simulink model "Flight_Test_Augmented_Model"  (R2024a)
settings: Solver=VariableStepAuto  StartTime=0.0  StopTime=55  RelTol=1e-3
undefined symbols (not defined in the file): a_e_tilde_hat_0, a_e_tilde_max, A_p, B_p, B_pT, degradation_switch, epsilon, g, Gamma_a, K_omega, K_p, k_r, K_v, L, Lambda_baseline, Lambda_deg, lambda_hat_0, lambda_max, nu_b_0, Omega_r_0, p_b_i_0, q_0, t_deg, T_max, T_min, tPoints, UAV, wind_switch, x_hat_0
libraries: matrix_library x2, shareduavrstlib x1
settings Model: Creator=Usuario  LastModifiedBy=Usuario

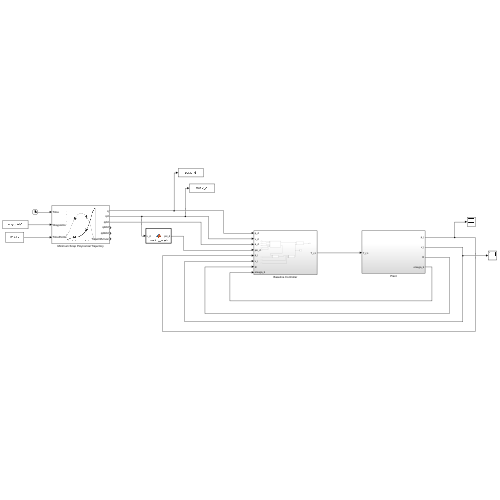
[thumbnail: Simulink's stored preview of the top-level diagram]
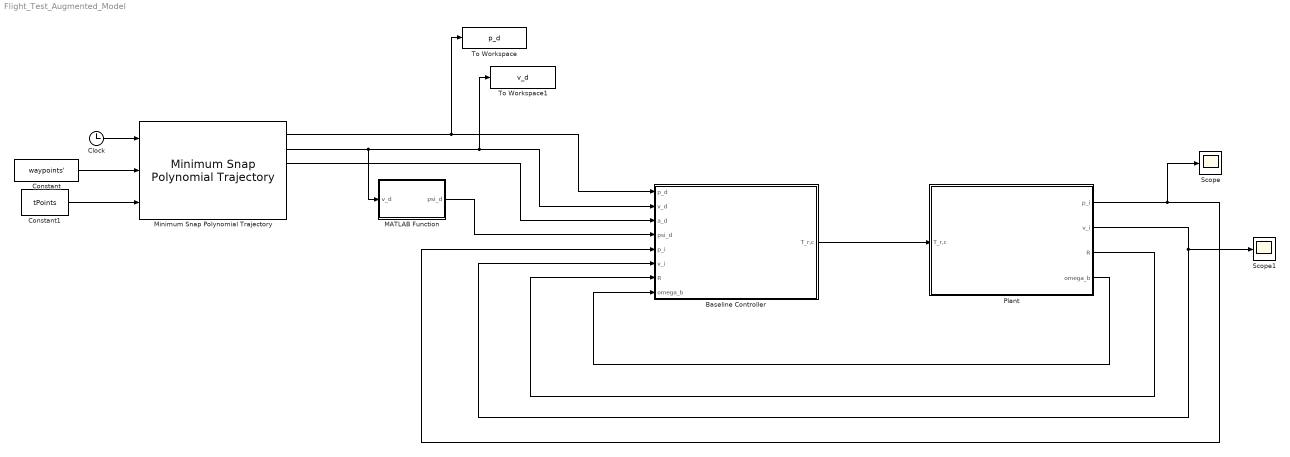
== system Flight_Test_Augmented_Model ==
  Baseline Controller : Subsystem
  Clock : Clock
  Constant : Constant  Value=waypoints'
  Constant1 : Constant  Value=tPoints
  MATLAB Function : MATLAB Function  TreatAsAtomicUnit=on
  Minimum Snap Polynomial Trajectory : shareduavrstlib/Minimum Snap Polynomial Trajectory  ShowBCInputPort=off  ShowPolynomialCoefs=off  ShowStatusOutputPort=off  TimeAllocation=off  TimeWeight=100  MinSegmentTime=0.1  MaxSegmentTime=1  MaxIteration=1500  MaxTime=10  SimulateUsing=Interpreted execution
      settings: LibrarySourceBlock=uavalgslib/Minimum Snap Polynomial Trajectory
  Plant : Subsystem
  Scope : Scope
  Scope1 : Scope
  To Workspace : ToWorkspace  VariableName=p_d  SaveFormat=Timeseries  SampleTime=-1
  To Workspace1 : ToWorkspace  VariableName=v_d  SaveFormat=Timeseries  SampleTime=-1
  wires:
  Baseline Controller/1(T_r,c) -> Plant/1(T_r,c)
  Plant/1(p_i) -> Scope/1, Baseline Controller/5(p_i)
  Plant/2(v_i) -> Baseline Controller/6(v_i), Scope1/1
  Plant/3(R) -> Baseline Controller/7(R)
  Plant/4(omega_b) -> Baseline Controller/8(omega_b)
  Minimum Snap Polynomial Trajectory/3 -> Baseline Controller/3(a_d)
  Clock/1 -> Minimum Snap Polynomial Trajectory/1
  Minimum Snap Polynomial Trajectory/1 -> Baseline Controller/1(p_d), To Workspace/1
  MATLAB Function/1(psi_d) -> Baseline Controller/4(psi_d)
  Constant/1 -> Minimum Snap Polynomial Trajectory/2
  Constant1/1 -> Minimum Snap Polynomial Trajectory/3
  Minimum Snap Polynomial Trajectory/2 -> MATLAB Function/1(v_d), Baseline Controller/2(v_d), To Workspace1/1

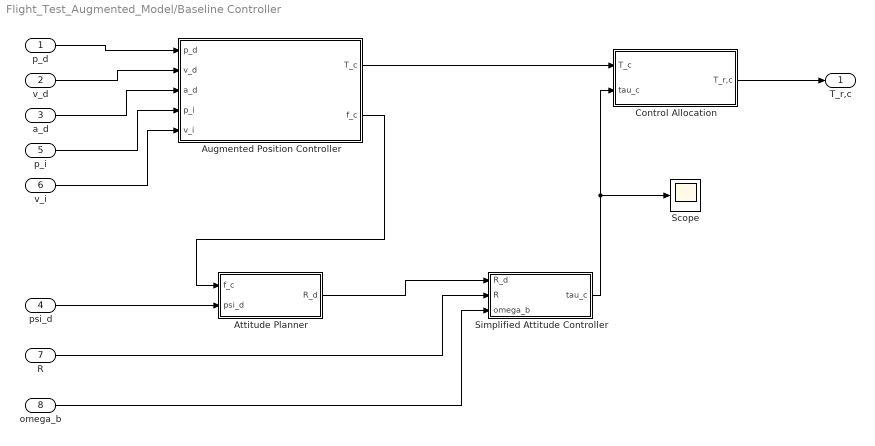
== system Flight_Test_Augmented_Model/Baseline Controller ==
  p_d : Inport
  v_d : Inport  Port=2
  a_d : Inport  Port=3
  psi_d : Inport  Port=4
  p_i : Inport  Port=5
  v_i : Inport  Port=6
  R : Inport  Port=7
  omega_b : Inport  Port=8
  Attitude Planner : Subsystem
  Augmented Position Controller : Subsystem
  Control Allocation : Subsystem
  Scope : Scope
  Simplified Attitude Controller : Subsystem
  T_r,c : Outport
  wires:
  Control Allocation/1(T_r,c) -> T_r,c/1
  p_d/1 -> Augmented Position Controller/1(p_d)
  v_d/1 -> Augmented Position Controller/2(v_d)
  a_d/1 -> Augmented Position Controller/3(a_d)
  Augmented Position Controller/1(T_c) -> Control Allocation/1(T_c)
  psi_d/1 -> Attitude Planner/2(psi_d)
  Augmented Position Controller/2(f_c) -> Attitude Planner/1(f_c)
  Attitude Planner/1(R_d) -> Simplified Attitude Controller/1(R_d)
  Simplified Attitude Controller/1(tau_c) -> Scope/1, Control Allocation/2(tau_c)
  p_i/1 -> Augmented Position Controller/4(p_i)
  v_i/1 -> Augmented Position Controller/5(v_i)
  R/1 -> Simplified Attitude Controller/2(R)
  omega_b/1 -> Simplified Attitude Controller/3(omega_b)

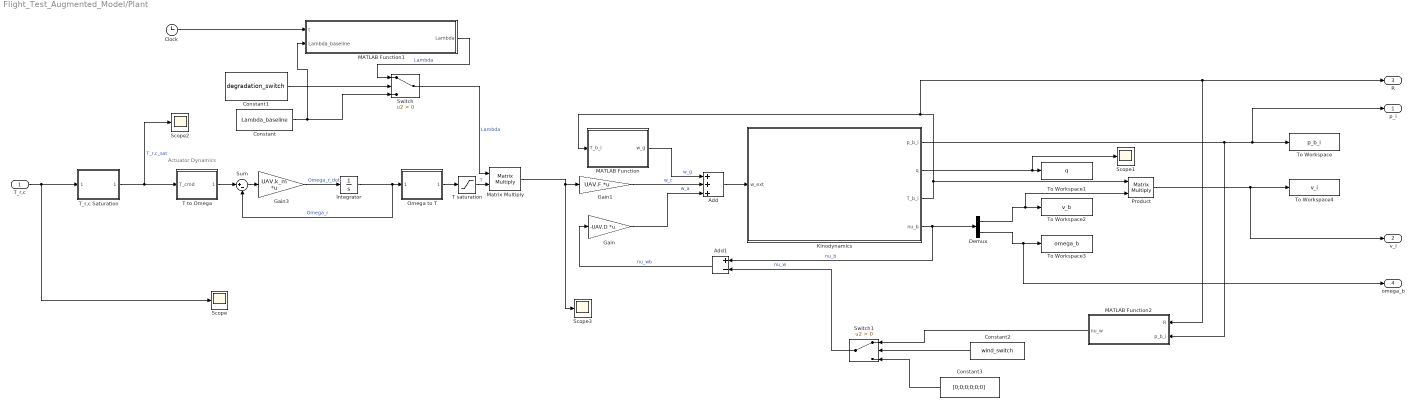
== system Flight_Test_Augmented_Model/Plant ==
  note: Actuator Dynamics
  T_r,c : Inport
  " Omega to T" : MATLAB Function  TreatAsAtomicUnit=on
  " T to Omega" : MATLAB Function  TreatAsAtomicUnit=on
  Add : Sum  Inputs=+++
  Add1 : Sum  Inputs=+-
  Clock : Clock
  Constant : Constant  Value=Lambda_baseline
  Constant1 : Constant  Value=degradation_switch
  Constant2 : Constant  Value=wind_switch
  Constant3 : Constant  Value=[0;0;0;0;0;0]
  Demux : Demux  Outputs=[3 3]
  Gain : Gain  Gain=-UAV.D  Multiplication=Matrix(K*u)
  Gain1 : Gain  Gain=UAV.F  Multiplication=Matrix(K*u)
  Gain3 : Gain  Gain=UAV.k_m  Multiplication=Matrix(K*u)
  Integrator : Integrator  InitialCondition=Omega_r_0
  Kinodynamics : Subsystem
  MATLAB Function : MATLAB Function  TreatAsAtomicUnit=on
  MATLAB Function1 : MATLAB Function  TreatAsAtomicUnit=on
  MATLAB Function2 : MATLAB Function  TreatAsAtomicUnit=on
  Matrix Multiply : Product  Multiplication=Matrix(*)
  Product : Product  Multiplication=Matrix(*)
  Scope{,1..3} (4 alike) : Scope
  Sum : Sum  Inputs=|+-
  Switch : Switch  Criteria=u2 > Threshold  SaturateOnIntegerOverflow=off  InputSameDT=off
  Switch1 : Switch  Criteria=u2 > Threshold  SaturateOnIntegerOverflow=off  InputSameDT=off
  T saturation : Saturate  UpperLimit=T_max  LowerLimit=T_min
  T_r,c Saturation : MATLAB Function  TreatAsAtomicUnit=on
  To Workspace : ToWorkspace  VariableName=p_b_i  SaveFormat=Timeseries  SampleTime=-1
  To Workspace1 : ToWorkspace  VariableName=q  SaveFormat=Timeseries  SampleTime=-1
  To Workspace2 : ToWorkspace  VariableName=v_b  SaveFormat=Timeseries  SampleTime=-1
  To Workspace3 : ToWorkspace  VariableName=omega_b  SaveFormat=Timeseries  SampleTime=-1
  To Workspace4 : ToWorkspace  VariableName=v_i  SaveFormat=Timeseries  SampleTime=-1
  p_i : Outport
  v_i : Outport  Port=2
  R : Outport  Port=3
  omega_b : Outport  Port=4
  wires:
  " T to Omega"/1(Omega_r_cmd) -> Sum/1
  Demux/2 -> omega_b/1, To Workspace3/1
  Add/1 -> Kinodynamics/1(w_ext)
  Kinodynamics/4(nu_b) -> Add1/1, Demux/1  "nu_b"
  Kinodynamics/2(q) -> Scope1/1, To Workspace1/1
  Product/1 -> v_i/1, To Workspace4/1
  Sum/1 -> Gain3/1
  Demux/1 -> Product/2, To Workspace2/1
  Gain/1 -> Add/3  "w_a"
  Gain1/1 -> Add/2  "w_c"
  Integrator/1 -> " Omega to T"/1(Omega_r), Sum/2  "Omega_r"
  MATLAB Function/1(w_g) -> Add/1  "w_g"
  Gain3/1 -> Integrator/1  "Omega_r_dot"
  T_r,c/1 -> T_r,c Saturation/1(Tr_cmd), Scope/1
  T_r,c Saturation/1(Tr_cmd_sat) -> Scope2/1, " T to Omega"/1(T_cmd)  "T_r,c_sat"
  " Omega to T"/1(T_ideal) -> T saturation/1
  T saturation/1 -> Matrix Multiply/2  "T"
  Matrix Multiply/1 -> Scope3/1, Gain1/1
  Constant/1 -> MATLAB Function1/2(Lambda_baseline), Switch/3
  Switch/1 -> Matrix Multiply/1  "Lambda"
  MATLAB Function1/1(Lambda) -> Switch/1  "Lambda"
  Constant1/1 -> Switch/2
  Clock/1 -> MATLAB Function1/1(t)
  Constant3/1 -> Switch1/3
  Kinodynamics/3(T_b_i) -> MATLAB Function2/1(R), R/1, MATLAB Function/1(T_b_i), Product/1
  Kinodynamics/1(p_b_i) -> MATLAB Function2/2(p_b_i), p_i/1, To Workspace/1
  Constant2/1 -> Switch1/2
  MATLAB Function2/1(nu_w) -> Switch1/1
  Switch1/1 -> Add1/2  "nu_w"
  Add1/1 -> Gain/1  "nu_wb"

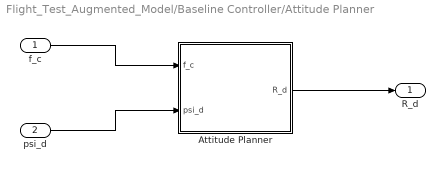
== system Flight_Test_Augmented_Model/Baseline Controller/Attitude Planner ==
  f_c : Inport
  psi_d : Inport  Port=2
  " Attitude Planner" : MATLAB Function  TreatAsAtomicUnit=on
  R_d : Outport
  wires:
  f_c/1 -> " Attitude Planner"/1(f_c)
  psi_d/1 -> " Attitude Planner"/2(psi_d)
  " Attitude Planner"/1(R_d) -> R_d/1

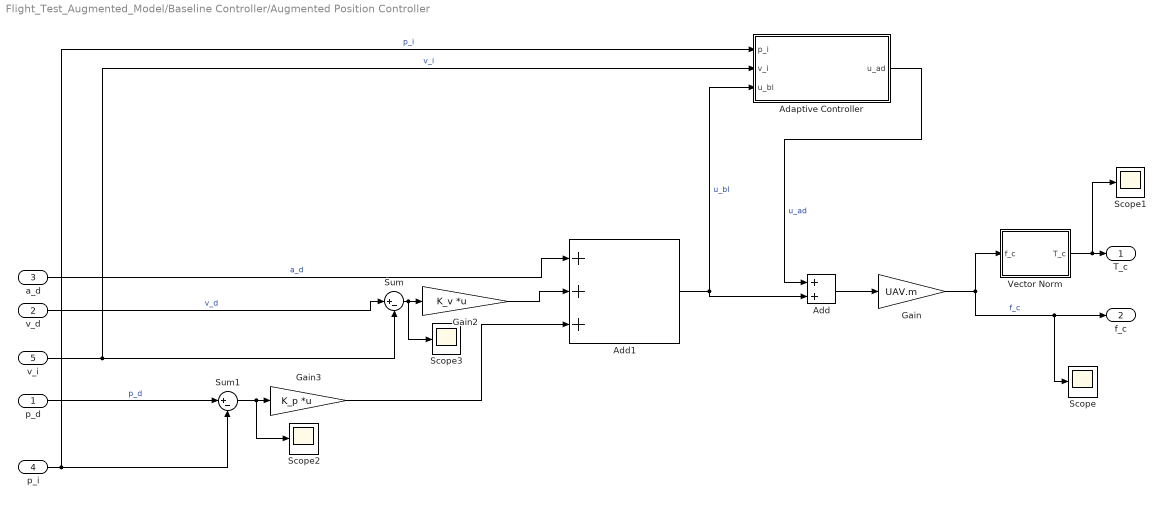
== system Flight_Test_Augmented_Model/Baseline Controller/Augmented Position Controller ==
  p_d : Inport
  v_d : Inport  Port=2
  a_d : Inport  Port=3
  p_i : Inport  Port=4
  v_i : Inport  Port=5
  Adaptive Controller : Subsystem
  Add : Sum
  Add1 : Sum  Inputs=+++
  Gain : Gain  Gain=UAV.m
  Gain2 : Gain  Gain=K_v  Multiplication=Matrix(K*u)
  Gain3 : Gain  Gain=K_p  Multiplication=Matrix(K*u)
  Scope{,1..3} (4 alike) : Scope
  Sum : Sum  Inputs=|+-
  Sum1 : Sum  Inputs=|+-
  Vector Norm : MATLAB Function  TreatAsAtomicUnit=on
  T_c : Outport
  f_c : Outport  Port=2
  wires:
  p_d/1 -> Sum1/1  "p_d"
  Gain3/1 -> Add1/3
  Sum1/1 -> Scope2/1, Gain3/1
  Sum/1 -> Scope3/1, Gain2/1
  a_d/1 -> Add1/1  "a_d"
  v_d/1 -> Sum/1  "v_d"
  p_i/1 -> Sum1/2, Adaptive Controller/1(p_i)  "p_i"
  v_i/1 -> Sum/2, Adaptive Controller/2(v_i)  "v_i"
  Gain/1 -> Vector Norm/1(f_c), Scope/1, f_c/1  "f_c"
  Vector Norm/1(T_c) -> Scope1/1, T_c/1
  Gain2/1 -> Add1/2
  Add/1 -> Gain/1
  Add1/1 -> Add/2, Adaptive Controller/3(u_bl)  "u_bl"
  Adaptive Controller/1(u_ad) -> Add/1  "u_ad"

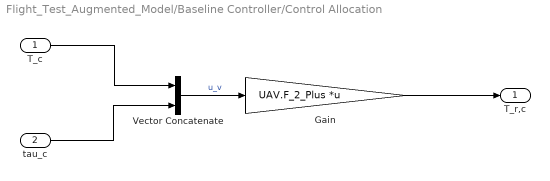
== system Flight_Test_Augmented_Model/Baseline Controller/Control Allocation ==
  T_c : Inport
  tau_c : Inport  Port=2
  Gain : Gain  Gain=UAV.F_2_Plus  Multiplication=Matrix(K*u)
  Vector Concatenate : Concatenate
  T_r,c : Outport
  wires:
  T_c/1 -> Vector Concatenate/1
  tau_c/1 -> Vector Concatenate/2
  Vector Concatenate/1 -> Gain/1  "u_v"
  Gain/1 -> T_r,c/1

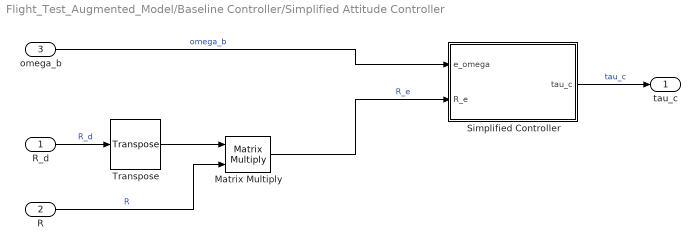
== system Flight_Test_Augmented_Model/Baseline Controller/Simplified Attitude Controller ==
  R_d : Inport
  R : Inport  Port=2
  omega_b : Inport  Port=3
  Matrix Multiply : Product  Multiplication=Matrix(*)
  Simplified Controller : MATLAB Function  TreatAsAtomicUnit=on
  Transpose : matrix_library/Transpose
  tau_c : Outport
  wires:
  omega_b/1 -> Simplified Controller/1(e_omega)  "omega_b"
  Matrix Multiply/1 -> Simplified Controller/2(R_e)  "R_e"
  Transpose/1 -> Matrix Multiply/1
  R_d/1 -> Transpose/1  "R_d"
  Simplified Controller/1(tau_c) -> tau_c/1  "tau_c"
  R/1 -> Matrix Multiply/2  "R"

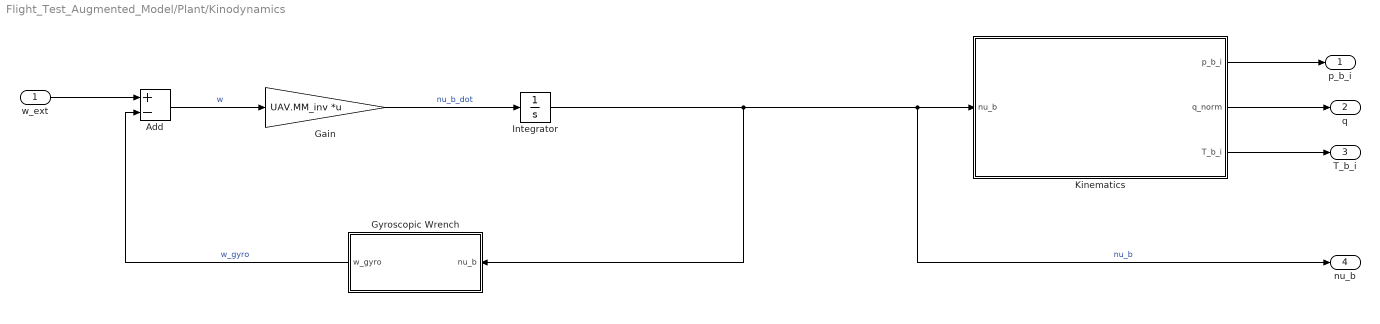
== system Flight_Test_Augmented_Model/Plant/Kinodynamics ==
  w_ext : Inport
  Add : Sum  Inputs=+-
  Gain : Gain  Gain=UAV.MM_inv  Multiplication=Matrix(K*u)
  Gyroscopic Wrench : MATLAB Function  TreatAsAtomicUnit=on
  Integrator : Integrator  InitialCondition=nu_b_0
  Kinematics : Subsystem
  p_b_i : Outport
  q : Outport  Port=2
  T_b_i : Outport  Port=3
  nu_b : Outport  Port=4
  wires:
  Kinematics/1(p_b_i) -> p_b_i/1
  w_ext/1 -> Add/1
  Integrator/1 -> Gyroscopic Wrench/1(nu_b), nu_b/1, Kinematics/1(nu_b)  "nu_b"
  Gain/1 -> Integrator/1  "nu_b_dot"
  Kinematics/3(T_b_i) -> T_b_i/1
  Kinematics/2(q_norm) -> q/1
  Gyroscopic Wrench/1(w_gyro) -> Add/2  "w_gyro"
  Add/1 -> Gain/1  "w"

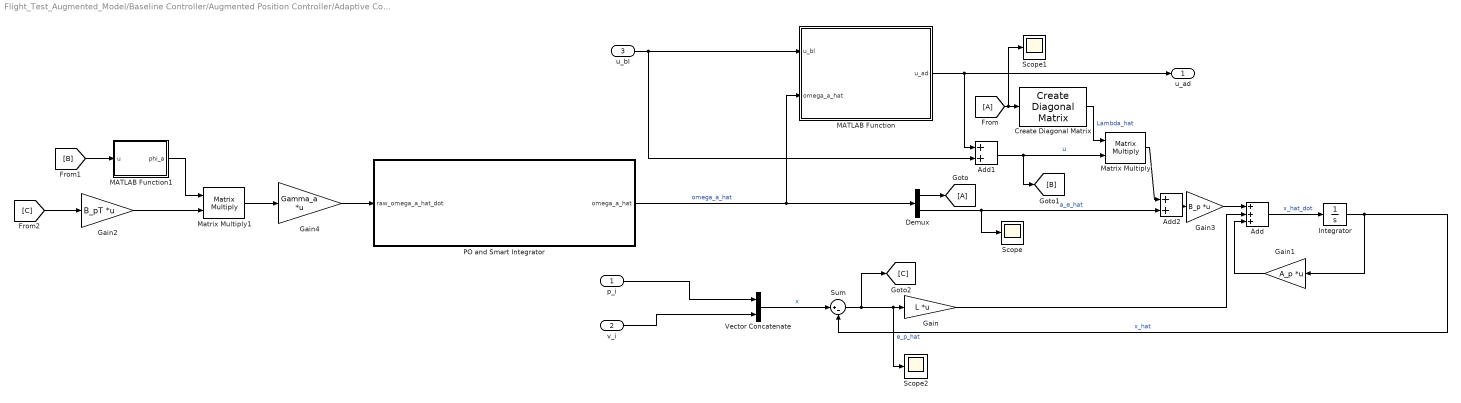
== system Flight_Test_Augmented_Model/Baseline Controller/Augmented Position Controller/Adaptive Controller ==
  p_i : Inport
  v_i : Inport  Port=2
  u_bl : Inport  Port=3
  Add : Sum  Inputs=+++
  Add1 : Sum
  Add2 : Sum
  Create Diagonal Matrix : matrix_library/Create Diagonal Matrix
      settings: LibrarySourceBlock=|
      | simulink/Matrix
      | Operations/Create Diagonal
      | Matrix
  Demux : Demux  Outputs=[3 3]
  From : From
  Gain : Gain  Gain=L  Multiplication=Matrix(K*u)
  Gain1 : Gain  Gain=A_p  Multiplication=Matrix(K*u)
  Gain2 : Gain  Gain=B_pT  Multiplication=Matrix(K*u)
  Gain3 : Gain  Gain=B_p  Multiplication=Matrix(K*u)
  Gain4 : Gain  Gain=Gamma_a  Multiplication=Matrix(K*u)
  Goto : Goto
  Integrator : Integrator  InitialCondition=x_hat_0
  MATLAB Function : MATLAB Function  TreatAsAtomicUnit=on
  MATLAB Function1 : MATLAB Function  TreatAsAtomicUnit=on
  Matrix Multiply : Product  Multiplication=Matrix(*)
  Matrix Multiply1 : Product  Multiplication=Matrix(*)
  PO and Smart Integrator : Subsystem
  Scope : Scope
  Scope1 : Scope
  Scope2 : Scope
  Sum : Sum  Inputs=|+-
  Vector Concatenate : Concatenate
  u_ad : Outport
  wires:
  u_bl/1 -> MATLAB Function/1(u_bl), Add1/2
  MATLAB Function/1(u_ad) -> Add1/1, u_ad/1
  Add/1 -> Integrator/1  "x_hat_dot"
  Integrator/1 -> Gain1/1, Sum/2  "x_hat"
  p_i/1 -> Vector Concatenate/1
  v_i/1 -> Vector Concatenate/2
  Vector Concatenate/1 -> Sum/1  "x"
  Sum/1 -> [C], Scope2/1, Gain/1  "e_p_hat"
  Gain/1 -> Add/2
  Gain1/1 -> Add/3
  Add2/1 -> Gain3/1
  Add1/1 -> [B], Matrix Multiply/2  "u"
  Create Diagonal Matrix/1 -> Matrix Multiply/1  "Lambda_hat"
  Matrix Multiply/1 -> Add2/1
  Demux/2 -> Scope/1, Add2/2  "a_e_hat"
  PO and Smart Integrator/1(omega_a_hat) -> MATLAB Function/2(omega_a_hat), Demux/1  "omega_a_hat"
  Demux/1 -> Goto/1
  From/1 -> Scope1/1, Create Diagonal Matrix/1
  Matrix Multiply1/1 -> Gain4/1
  [C] -> Gain2/1
  Gain2/1 -> Matrix Multiply1/2
  [B] -> MATLAB Function1/1(u)
  MATLAB Function1/1(phi_a) -> Matrix Multiply1/1
  Gain3/1 -> Add/1
  Gain4/1 -> PO and Smart Integrator/1(raw_omega_a_hat_dot)

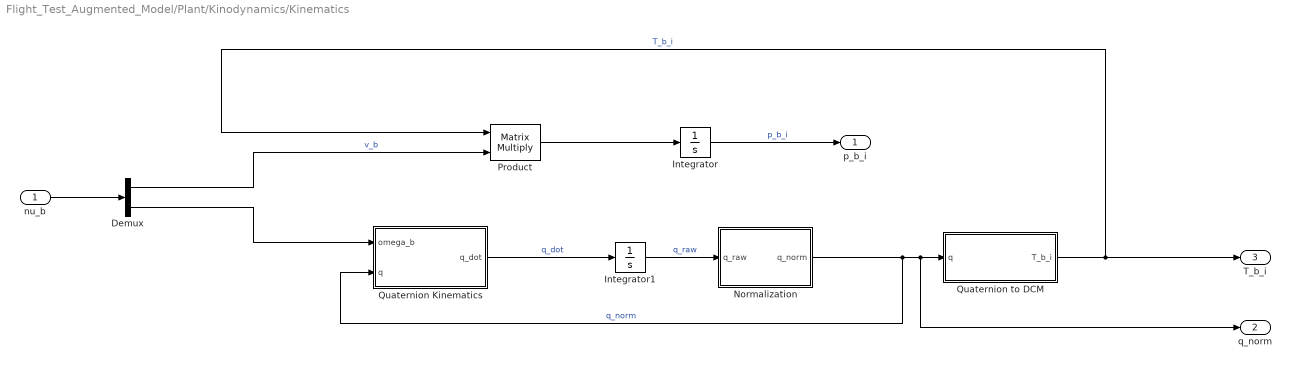
== system Flight_Test_Augmented_Model/Plant/Kinodynamics/Kinematics ==
  nu_b : Inport
  " Normalization" : MATLAB Function  TreatAsAtomicUnit=on
  Demux : Demux  Outputs=[3 3]
  Integrator : Integrator  InitialCondition=p_b_i_0
  Integrator1 : Integrator  InitialCondition=q_0
  Product : Product  Multiplication=Matrix(*)
  Quaternion Kinematics : MATLAB Function  TreatAsAtomicUnit=on
  Quaternion to DCM : MATLAB Function  TreatAsAtomicUnit=on
  p_b_i : Outport
  q_norm : Outport  Port=2
  T_b_i : Outport  Port=3
  wires:
  Integrator1/1 -> " Normalization"/1(q_raw)  "q_raw"
  " Normalization"/1(q_norm) -> Quaternion to DCM/1(q), q_norm/1, Quaternion Kinematics/2(q)  "q_norm"
  Demux/2 -> Quaternion Kinematics/1(omega_b)
  Quaternion Kinematics/1(q_dot) -> Integrator1/1  "q_dot"
  Product/1 -> Integrator/1
  Quaternion to DCM/1(T_b_i) -> T_b_i/1, Product/1  "T_b_i"
  Demux/1 -> Product/2  "v_b"
  Integrator/1 -> p_b_i/1  "p_b_i"
  nu_b/1 -> Demux/1

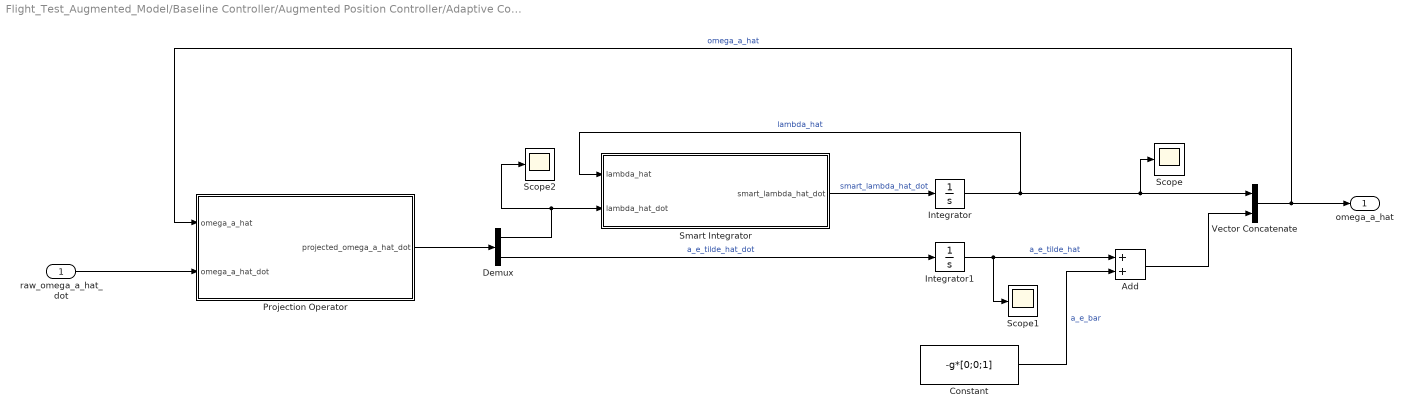
== system Flight_Test_Augmented_Model/Baseline Controller/Augmented Position Controller/Adaptive Controller/PO and Smart Integrator ==
  raw_omega_a_hat_dot : Inport
  " Smart Integrator" : MATLAB Function  TreatAsAtomicUnit=on
  Add : Sum
  Constant : Constant  Value=-g*[0;0;1]
  Demux : Demux  Outputs=[3 3]
  Integrator : Integrator  InitialCondition=lambda_hat_0
  Integrator1 : Integrator  InitialCondition=a_e_tilde_hat_0
  Projection Operator : MATLAB Function  TreatAsAtomicUnit=on
  Scope : Scope
  Scope1 : Scope
  Scope2 : Scope
  Vector Concatenate : Concatenate
  omega_a_hat : Outport
  wires:
  Integrator1/1 -> Scope1/1, Add/1  "a_e_tilde_hat"
  Demux/2 -> Integrator1/1  "a_e_tilde_hat_dot"
  Constant/1 -> Add/2  "a_e_bar"
  Integrator/1 -> " Smart Integrator"/1(lambda_hat), Scope/1, Vector Concatenate/1  "lambda_hat"
  " Smart Integrator"/1(smart_lambda_hat_dot) -> Integrator/1  "smart_lambda_hat_dot"
  Add/1 -> Vector Concatenate/2
  Vector Concatenate/1 -> Projection Operator/1(omega_a_hat), omega_a_hat/1  "omega_a_hat"
  Demux/1 -> Scope2/1, " Smart Integrator"/2(lambda_hat_dot)
  Projection Operator/1(projected_omega_a_hat_dot) -> Demux/1
  raw_omega_a_hat_dot/1 -> Projection Operator/2(omega_a_hat_dot)

== matlab function Flight_Test_Augmented_Model/Baseline Controller/Augmented Position Controller/Adaptive Controller/MATLAB Function ==
  data: u_bl input; omega_a_hat input; u_ad output
function u_ad=adaptive_control_input(u_bl,omega_a_hat)
Lambda_hat=diag(omega_a_hat(1:3));
a_e_hat=omega_a_hat(4:6);

u_ad=(Lambda_hat\u_bl-u_bl)-Lambda_hat\a_e_hat;
end

== matlab function Flight_Test_Augmented_Model/Baseline Controller/Augmented Position Controller/Adaptive Controller/MATLAB Function1 ==
  data: u input; phi_a output
function phi_a=construct_phi_a(u)
%This function constructs phi_a for the given augmentation problem. 
phi_a=[diag(u);eye(3,3)];
end

== matlab function Flight_Test_Augmented_Model/Baseline Controller/Augmented Position Controller/Adaptive Controller/PO and Smart Integrator/ Smart Integrator ==
  data: lambda_hat input; lambda_hat_dot input; smart_lambda_hat_dot output; lambda_min parameter
function smart_lambda_hat_dot=smart_integrator(lambda_hat,lambda_hat_dot,lambda_min)
%This function is a smart integrator designed to avoid lambda terms going
%to zero,  making the Lambda matrix singular and blowing up the algorithm. 
smart_lambda_hat_dot=nan(3,1);

%It's not completely impervious, since it would need an event detector and
%so on, but it should be enough for the problem at hand. 
for i=1:3
    if lambda_hat(i)>lambda_min
        smart_lambda_hat_dot(i)=lambda_hat_dot(i);
    elseif lambda_hat_dot(i)>=0
        smart_lambda_hat_dot(i)=lambda_hat_dot(i);
    else
        smart_lambda_hat_dot(i)=0;
    end
end

end

== matlab function Flight_Test_Augmented_Model/Plant/Kinodynamics/Kinematics/Quaternion to DCM ==
  data: q input; T_b_i output
function T_b_i=quaternion_to_DCM(q)
%My implementation of the quaternion to DCM transformation, to ensure
%consistency. It must return the active representation of the rotation
%between i and b, which will be the DCM from b to i. 
eta=q(1);
epsilon=q(2:4);
epsilon_x=cross_matrix(epsilon);

T_b_i=eye(3,3)+2*eta*epsilon_x+2*epsilon_x*epsilon_x;
end

== matlab function Flight_Test_Augmented_Model/Baseline Controller/Augmented Position Controller/Adaptive Controller/PO and Smart Integrator/Projection Operator ==
  data: omega_a_hat input; projected_omega_a_hat_dot output; omega_a_hat_dot input; epsilon parameter; lambda_max parameter; a_e_tilde_max parameter
function projected_omega_a_hat_dot=PO(omega_a_hat,omega_a_hat_dot,epsilon, lambda_max, a_e_tilde_max)
%This function applies the projection operator to the adaptive laws, to
%ensure a robust implementation. The first three components of omega_hat_a,
%related to the lambda vector, are each bounded individually. The last
%three are bounded in unison but with an offset according to the gravity
%vector in inertial frame. 
projected_omega_a_hat_dot=nan(6,1);
%Apply PO to each component of lambda: 
for i=1:3
    %Construct f and df
    f=((1+epsilon)*omega_a_hat(i)^2-lambda_max^2)/(epsilon*lambda_max^2);
    df=2*(1+epsilon)/(epsilon*lambda_max^2)*omega_a_hat(i);
    
    %Check which case is applicable: 
    if f>0 && df*omega_a_hat_dot(i)>0
        projected_omega_a_hat_dot(i)=(1-f)*omega_a_hat_dot(i); %simplifies in the scalar case 
    else
        projected_omega_a_hat_dot(i)=omega_a_hat_dot(i);
    end
end
%Apply PO to a_e_tilde: 
f=((1+epsilon)*omega_a_hat(4:6)'*omega_a_hat(4:6)-a_e_tilde_max^2)/(epsilon*a_e_tilde_max^2);
gradf=2*(1+epsilon)/(epsilon*a_e_tilde_max^2)*omega_a_hat(4:6);

if f>0 && gradf'*omega_a_hat_dot(4:6)>0
    projected_omega_a_hat_dot(4:6)=omega_a_hat_dot(4:6)-f*(gradf*gradf')*omega_a_hat_dot(4:6)/(gradf'*gradf);
else
    projected_omega_a_hat_dot(4:6)=omega_a_hat_dot(4:6);
end
end

== matlab function Flight_Test_Augmented_Model/Plant/MATLAB Function1 ==
  data: t input; Lambda output; Lambda_baseline input; t_deg parameter; Lambda_deg parameter
function Lambda=Effectiveness_model(t,Lambda_baseline,t_deg, Lambda_deg)
%this function allows the modelling of a sudden degradation in the control
%effectiveness at time t_deg to Lambda_deg.
if t<t_deg
    Lambda=Lambda_baseline;
else
    Lambda=Lambda_deg;
end
end

== matlab function Flight_Test_Augmented_Model/Plant/MATLAB Function2 ==
  data: nu_w output; R input; p_b_i input; w_intensity parameter
function nu_w=wind_velocity(R,p_b_i,w_intensity)
%This function will introduce a specified wind velocity between the first
%and second line of buildings, in the inertial y direction. 
if p_b_i(2)<=0 && p_b_i(2)>=-20
    v_w_i=w_intensity*[0;1;0];
    nu_w=[R'*v_w_i;zeros(3,1)];
else
    nu_w=zeros(6,1);
end
end

== matlab function Flight_Test_Augmented_Model/Plant/Kinodynamics/Kinematics/ Normalization ==
  data: q_raw input; q_norm output
function q_norm=normalization(q_raw)

q_norm=q_raw/norm(q_raw);

== matlab function Flight_Test_Augmented_Model/Plant/Kinodynamics/Kinematics/Quaternion Kinematics ==
  data: omega_b input; q_dot output; q input
function q_dot = quat_kinematics(omega_b,q)
%Quaternion kinematics. Requires that omega_b be a column vector. q must
%also be a column vector following the course's quaternion convention. 
eta=q(1);
epsilon=q(2:4);
epsilon_x=cross_matrix(epsilon);

q_dot=1/2*[-epsilon';epsilon_x+eta*eye(3,3)]*omega_b;
end

== matlab function Flight_Test_Augmented_Model/Plant/Kinodynamics/Gyroscopic Wrench ==
  data: nu_b input; w_gyro output; UAV parameter
function w_gyro=gyroscopic_wrench(nu_b,UAV)
nu_b_southwest=[cross_matrix(nu_b(4:6)),zeros(3,3);cross_matrix(nu_b(1:3)),cross_matrix(nu_b(4:6))];
w_gyro=nu_b_southwest*UAV.MM*nu_b;
end

== matlab function Flight_Test_Augmented_Model/Plant/MATLAB Function ==
  data: T_b_i input; w_g output; UAV parameter; g parameter
function w_g=Gravity_Wrench(T_b_i,UAV, g)
e3=[0;0;1];

w_g=-g*[UAV.m*T_b_i'*e3;UAV.S_t*T_b_i'*e3];
end

== matlab function Flight_Test_Augmented_Model/Plant/ T to Omega ==
  data: T_cmd input; Omega_r_cmd output; k_f parameter
function Omega_r_cmd=T_to_Omega(T_cmd,k_f)
Omega_r_cmd=sqrt(T_cmd/k_f);
end

== matlab function Flight_Test_Augmented_Model/Plant/ Omega to T ==
  data: Omega_r input; T_ideal output; k_f parameter
function T_ideal=Omega_to_T(Omega_r,k_f)
T_ideal=k_f*Omega_r.^2;
end

== matlab function Flight_Test_Augmented_Model/MATLAB Function ==
  data: v_d input; psi_d output
function psi_d=heading_angle(v_d)
%This function computes the heading angle necessary to keep the UAV aligned
%with the trajectory. 
psi_d=atan2(v_d(2),v_d(1)); %arctan(vy/vx), with 4 quadrants
end

== matlab function Flight_Test_Augmented_Model/Baseline Controller/Augmented Position Controller/Vector Norm ==
  data: f_c input; T_c output
function T_c=norm(f_c)
T_c=norm(f_c);
end

== matlab function Flight_Test_Augmented_Model/Baseline Controller/Attitude Planner/ Attitude Planner ==
  data: f_c input; R_d output; psi_d input
function R_d=Attitude_Planner(f_c,psi_d)
%This function implements the attitude planner logic in P2CS1. It
%constructs the expression of the basis vectors of the desired attitude in 
%the inertial frame and uses them to construct R_d. For details, see slides.  
k_p_i=f_c/norm(f_c);
h_d_i=[cos(psi_d);sin(psi_d);0];
j_p_i=cross(k_p_i,h_d_i)/norm(cross(k_p_i,h_d_i));
i_p_i=cross(j_p_i,k_p_i)/norm(cross(j_p_i,k_p_i)); %normalization not necessary in theory, but I implement it just in case there are some numerical errors.

R_d=[i_p_i,j_p_i,k_p_i];
end

== matlab function Flight_Test_Augmented_Model/Plant/T_r,c Saturation ==
  data: Tr_cmd input; Tr_cmd_sat output; T_min parameter; T_max parameter
function Tr_cmd_sat=Command_Input_Saturation(Tr_cmd,T_min, T_max)
Tr_cmd_sat=nan(size(Tr_cmd));
for i=1:length(Tr_cmd)
    if Tr_cmd(i)<T_min
        Tr_cmd_sat(i)=T_min;
    elseif Tr_cmd(i)>T_max
        Tr_cmd_sat(i)=T_max;
    else
        Tr_cmd_sat(i)=Tr_cmd(i);
    end
end
end

== matlab function Flight_Test_Augmented_Model/Baseline Controller/Simplified Attitude Controller/Simplified Controller ==
  data: e_omega input; tau_c output; R_e input; k_r parameter; K_omega parameter
function tau_c=Controller(e_omega,R_e,k_r, K_omega)
%Construct er
e_r=zeros(3,1);
I=eye(3,3);
for i=1:3
    e_r=e_r+k_r(i)*cross_matrix(R_e'*I(:,i))*I(:,i);
end
%Construct tau_c
tau_c=-e_r-K_omega*e_omega;

end
